simulink model "model45V"  (R2020b)
settings: Solver=VariableStepAuto  StartTime=0.0  StopTime=1  RelTol=1e-3
settings Model: Creator=anton  LastModifiedBy=anton

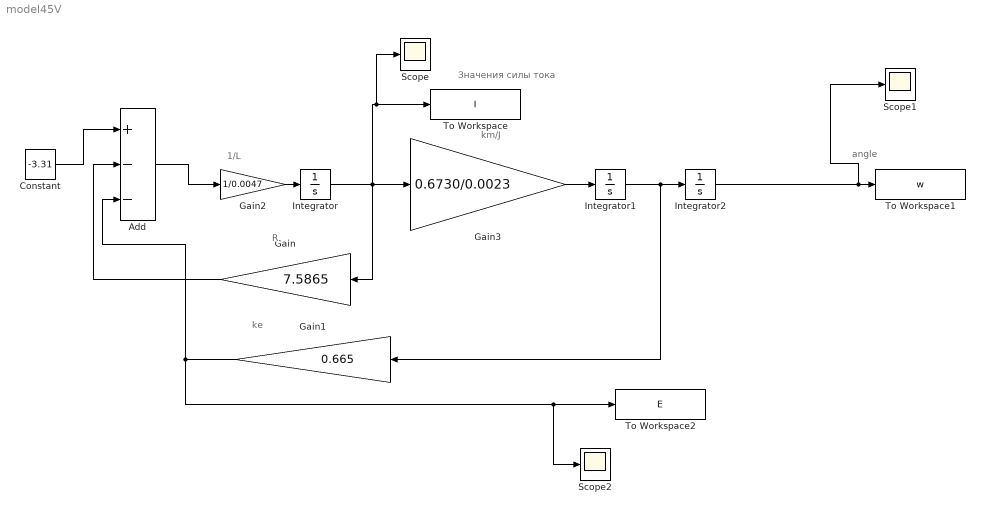
== system model45V ==
  note: km/J
  note: R
  note: ke
  note: 1/L
  note: angle
  note: Значения силы тока
  Add : Sum  Inputs=+--
  Constant : Constant  Value=-3.31  SampleTime=-1
  Gain : Gain  Gain=7.5865
  Gain1 : Gain  Gain=0.665
  Gain2 : Gain  Gain=1/0.0047
  Gain3 : Gain  Gain=0.6730/0.0023
  Integrator : Integrator
  Integrator1 : Integrator
  Integrator2 : Integrator
  Scope : Scope
  Scope1 : Scope
  Scope2 : Scope
  To Workspace : ToWorkspace  VariableName=I  SaveFormat=Timeseries  SampleTime=-1
  To Workspace1 : ToWorkspace  VariableName=w  SaveFormat=Timeseries  SampleTime=-1
  To Workspace2 : ToWorkspace  VariableName=E  SaveFormat=Timeseries  SampleTime=-1
  wires:
  Constant/1 -> Add/1
  Gain/1 -> Add/2
  Gain1/1 -> Add/3, Scope2/1, To Workspace2/1
  Add/1 -> Gain2/1
  Gain2/1 -> Integrator/1
  Integrator/1 -> Gain/1, Gain3/1, To Workspace/1, Scope/1
  Gain3/1 -> Integrator1/1
  Integrator1/1 -> Gain1/1, Integrator2/1
  Integrator2/1 -> Scope1/1, To Workspace1/1
